simulink model "linnovi"  (R2020b)
settings: Solver=VariableStepAuto  StartTime=0.0  StopTime=10.0  RelTol=1e-3
values from neighbouring files (symbols this model uses):
  b1 = 0.0050134512    [I_PD.m]    (also in LQR.m = 0.05; PODACI.m = 0.05; Untitled2.m)
  b2 = 45    [LQR.m]    (also in PODACI.m)
  c = 0.03    [LQR.m]    (also in PODACI.m)
  d = 0.062    [LQR.m]    (also in PODACI.m)
  g = 9.81    [LQR.m]    (also in PODACI.m)
  M = 1.2    [LQR.m]    (also in PODACI.m)
  m = 0.3    [LQR.m]    (also in PODACI.m)
settings Model: Creator=Toni  LastModifiedBy=Toni

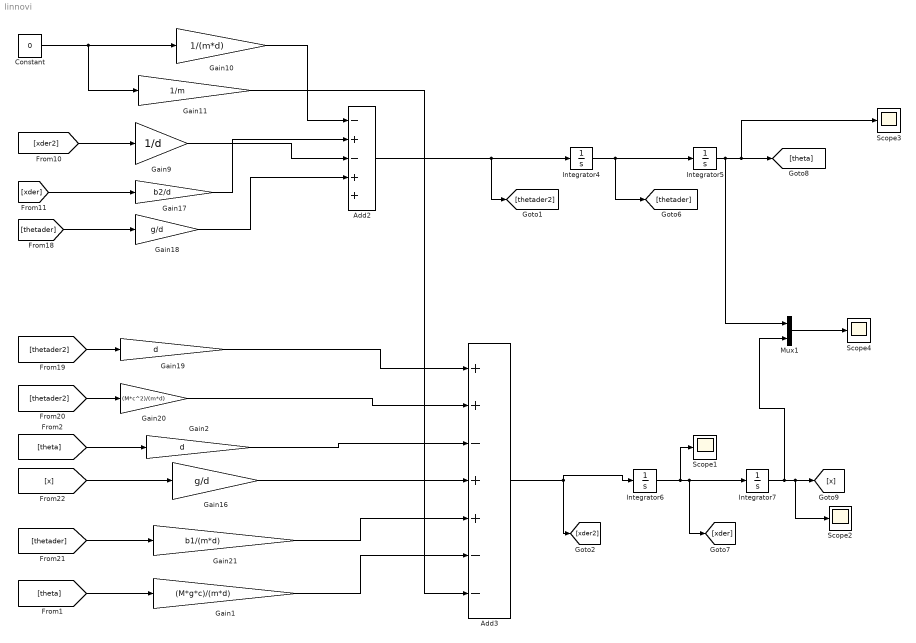
== system linnovi ==
  Add2 : Sum  Inputs=-+-++
  Add3 : Sum  Inputs=++-++--
  Constant : Constant  Value=0
  Gain1 : Gain  Gain=(M*g*c)/(m*d)
  Gain10 : Gain  Gain=1/(m*d)
  Gain11 : Gain  Gain=1/m
  Gain16 : Gain  Gain=g/d
  Gain17 : Gain  Gain=b2/d
  Gain18 : Gain  Gain=g/d
  Gain19 : Gain  Gain=d
  Gain2 : Gain  Gain=d
  Gain20 : Gain  Gain=(M*c^2)/(m*d)
  Gain21 : Gain  Gain=b1/(m*d)
  Gain9 : Gain  Gain=1/d
  Integrator{4..7} (4 alike) : Integrator
  Mux1 : Mux  Inputs=2
  Scope{1..4} (4 alike) : Scope
  wires:
  Constant/1 -> Gain10/1, Gain11/1
  [xder2] -> Gain9/1
  [xder] -> Gain17/1
  Add2/1 -> [thetader2], Integrator4/1
  [thetader2] -> Gain20/1
  [thetader] -> Gain21/1
  Gain19/1 -> Add3/1
  Gain20/1 -> Add3/2
  Gain18/1 -> Add2/4
  Integrator5/1 -> [theta], Scope3/1, Mux1/1
  [thetader2] -> Gain19/1
  Gain17/1 -> Add2/2
  [thetader] -> Gain18/1
  Integrator7/1 -> Mux1/2, Scope2/1, [x]
  Gain16/1 -> Add3/4
  Integrator4/1 -> Integrator5/1, [thetader]
  Gain11/1 -> Add3/7
  Integrator6/1 -> Scope1/1, Integrator7/1, [xder]
  Mux1/1 -> Scope4/1
  Gain10/1 -> Add2/1
  Add3/1 -> [xder2], Integrator6/1
  Gain21/1 -> Add3/5
  [x] -> Gain16/1
  Gain9/1 -> Add2/3
  [theta] -> Gain1/1
  Gain1/1 -> Add3/6
  [theta] -> Gain2/1
  Gain2/1 -> Add3/3
